simulink model "Projectile-Trajectory-Simulation"  (R2024b)
settings: Solver=VariableStepAuto  StartTime=0.0  StopTime=2  RelTol=1e-3
undefined symbols (not defined in the file): Cd, g, m, rho
settings Model: Creator=nafis  LastModifiedBy=nafis
settings SolverCC: DateTimeAtSimulationTimeZero=[]

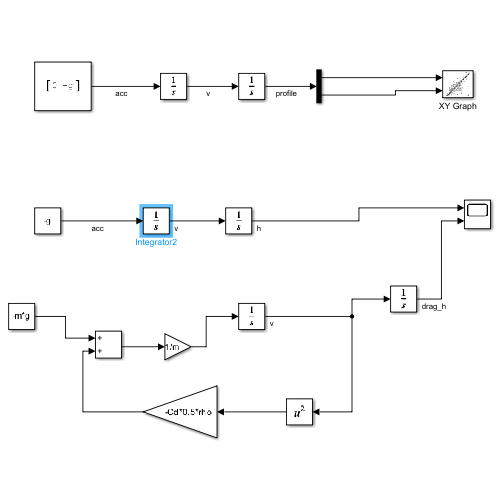
[thumbnail: Simulink's stored preview of the top-level diagram]
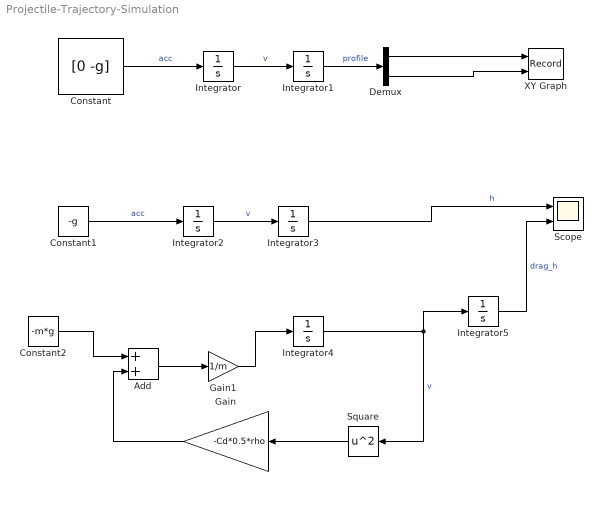
== system Projectile-Trajectory-Simulation ==
  Add : Sum
  Constant : Constant  Value=[0 -g]
  Constant1 : Constant  Value=-g
  Constant2 : Constant  Value=-m*g
  Demux : Demux  Outputs=2
  Gain : Gain  Gain=-Cd*0.5*rho
  Gain1 : Gain  Gain=1/m
  Integrator : Integrator  InitialCondition=[100*cos(45) 100*sin(45)]
  Integrator1 : Integrator
  Integrator2 : Integrator  InitialCondition=100*sin(45)
  Integrator3 : Integrator
  Integrator4 : Integrator  InitialCondition=100*sin(45)
  Integrator5 : Integrator
  Scope : Scope  NumInputPorts=2
  Square : Math  Operator=square
  XY Graph : Record  FileSettingsInternal="{\"entries\":[{\"content\":{\"excelSettings\":{\"content\":{},\"type\":\"Streamout.ExcelSettings\"}},\"type\":\"Streamout.FileSettingStorage\",\"uuid\":\"\"}],\"packageUris\":[\"http:\\/\\/schema.mathworks.com\\/mf0\\/streamout_blocks\\/R2020a\"],\"version\":\"1.0\"}"  Layout=[1 1]  SignalsInternal="{\"entries\":[{\"content\":{\"signals\":[{\"content\":{\"blockPath\":[],\"dimensions\":[1],\"domain\":\"\",\"lineColor\":\"#a2142f\",\"plots\":[ 1 ],\"port\":1,\"sid\":[\"\"],\"signalID\":1,\"signalName\":\"Demux:1\"},\"type\":\"RecordBlkView.Signal\",\"uuid\":\"\"},{\"content\":{\"blockPath\":[],\"dimensions\":[1],\"domain\":\"\",\"lineColor\":\"#139fff\",\"plots\":[ 1 ],\"port\":2,\"sid\":[\"\"],\"signalID\":2,\"signalName\":\"Demux:2\"},\"type\":\"RecordBlkView.Signal\",\"uuid\":\"\"}]},\"type\":\"RecordBlkView.InputSignals\",\"uuid\":\"\"}],\"packageUris\":[\"http:\\/\\/schema.mathworks.com\\/mf0\\/streamout_blocks\\/R2020a\"],\"version\":\"1.0\"}"  VisualizationBindings="{\"xyplotplugin\":{\"info\":[{\"series\":[{\"bindingParametersList\":[{\"parameter\":\"X-Axis\",\"signalID\":1,\"signalName\":\"Demux:1\"},{\"parameter\":\"Y-Axis\",\"signalID\":2,\"signalName\":\"Demux:2\"}],\"seriesID\":0}],\"subplotID\":1}]}}"  CompatibilityTag=XY
  wires:
  Constant/1 -> Integrator/1  "acc"
  Integrator/1 -> Integrator1/1  "v"
  Integrator1/1 -> Demux/1  "profile"
  Demux/1 -> XY Graph/1
  Demux/2 -> XY Graph/2
  Constant1/1 -> Integrator2/1  "acc"
  Integrator2/1 -> Integrator3/1  "v"
  Integrator3/1 -> Scope/1  "h"
  Integrator4/1 -> Square/1, Integrator5/1  "v"
  Constant2/1 -> Add/1
  Add/1 -> Gain1/1
  Gain1/1 -> Integrator4/1
  Integrator5/1 -> Scope/2  "drag_h"
  Square/1 -> Gain/1
  Gain/1 -> Add/2
